simulink model "A1_p2_4_sim"  (R2019a)
settings: Solver=VariableStepAuto  StartTime=0.0  StopTime=10.0  RelTol=1e-3
values from neighbouring files (symbols this model uses):
  k_d = 1    [A1_p2_4.m]    (also in problem2_4.m = 0.02)
  k_i = 0.1    [A1_p2_4.m]    (also in problem2_4.m = 5e-08)
  k_p = 1    [A1_p2_4.m]    (also in problem2_4.m = 5e-05)
settings Model: Creator=paalthorseth  LastModifiedBy=paalthorseth

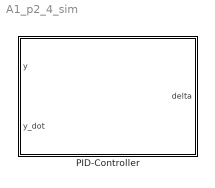
== system A1_p2_4_sim ==
  PID-Controller : Subsystem

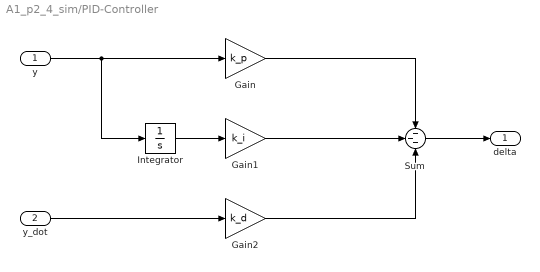
== system A1_p2_4_sim/PID-Controller ==
  y : Inport
  y_dot : Inport  Port=2
  Gain : Gain  Gain=k_p
  Gain1 : Gain  Gain=k_i
  Gain2 : Gain  Gain=k_d
  Integrator : Integrator
  Sum : Sum  Inputs=---
  delta : Outport
  wires:
  Sum/1 -> delta/1
  y_dot/1 -> Gain2/1
  Integrator/1 -> Gain1/1
  Gain/1 -> Sum/1
  Gain1/1 -> Sum/2
  Gain2/1 -> Sum/3
  y/1 -> Integrator/1, Gain/1
